simulink model "mrac_sim"  (R2023b)
settings: Solver=VariableStepAuto  StartTime=0.0  StopTime=2200  FixedStep=0.1  RelTol=1e-3  EnableMultiTasking=on
settings Model: Creator=Admin  LastModifiedBy=andre
settings SolverCC: AlgebraicLoopSolver=TrustRegion
settings DataIOCC: LimitDataPoints=on  SaveFormat=Array  ReturnWorkspaceOutputs=off
settings OptimizationCC: ReuseModelBlockBuffer=off  LifeSpan=inf
settings DebuggingCC: UnconnectedInputMsg=warning  UnconnectedOutputMsg=warning  UnconnectedLineMsg=warning  SFUnexpectedBacktrackingDiag=warning  SFNoUnconditionalDefaultTransitionDiag=warning  SFExecutionAtInitializationDiag=none  ArithmeticOperatorsInVariantConditions=warning
settings HardwareCC: ProdBitPerPointer=32  ProdBitPerSizeT=32  ProdBitPerPtrDiffT=32  ProdLargestAtomicFloat=None  ProdIntDivRoundTo=Undefined  ProdEndianess=Unspecified  ProdWordSize=32  ProdHWDeviceType=32-bit Generic
settings ModelReferenceCC: PropagateSignalLabelsOutOfModel=off
settings SFSimCC: SimUseLocalCustomCode=off  CustomCodeUndefinedFunction=UseInterfaceOnly
settings RTWCC: RTWUseLocalCustomCode=off
settings CodeAppCC: StateflowObjectComments=on
settings GRTTargetCC: TargetLangStandard=C89/C90 (ANSI)
settings ConfigComp: CovMetricSettings=dw  CovSaveCumulativeToWorkspaceVar=on  CovSaveSingleToWorkspaceVar=on  CovExternalEMLEnable=off

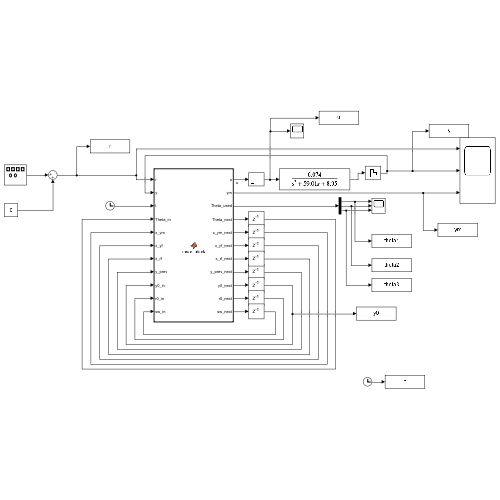
[thumbnail: Simulink's stored preview of the top-level diagram]
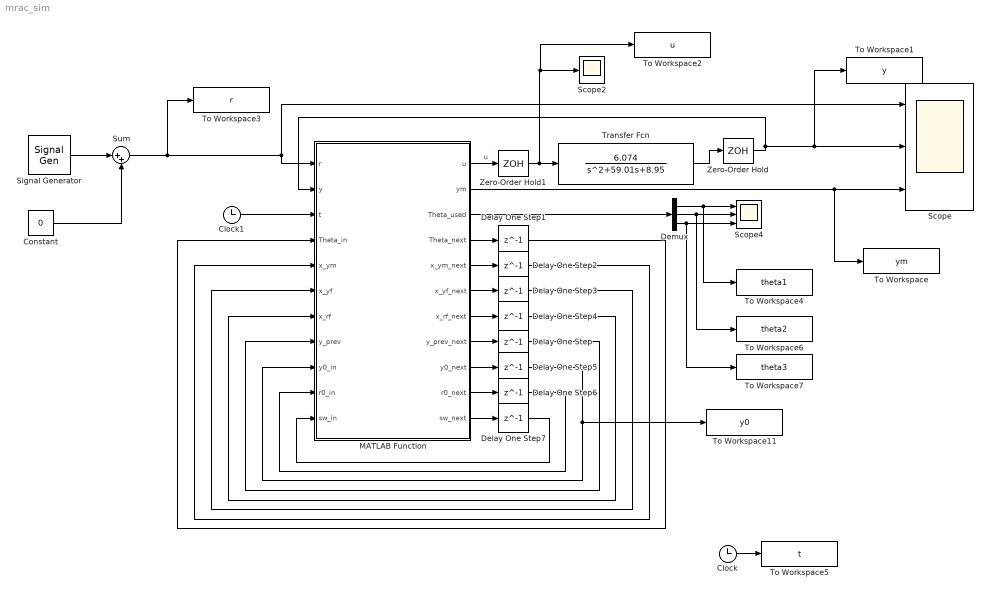
== system mrac_sim ==
  Clock : Clock
  Clock1 : Clock
  Constant : Constant  Value=0
  Delay One Step{,1..7} (8 alike) : Delay  DelayLength=1
  Demux : Demux  Outputs=3
  MATLAB Function : MATLAB Function  TreatAsAtomicUnit=on
  Scope : Scope  NumInputPorts=3
  Scope2 : Scope
  Scope4 : Scope  NumInputPorts=3
  Signal Generator : SignalGenerator  Amplitude=0.5  Frequency=1/400
  Sum : Sum  Inputs=|++
  To Workspace : ToWorkspace  VariableName=ym  SampleTime=0.1
      settings: Save2DSignal=2-D array (concatenate along first dimension)
  To Workspace1 : ToWorkspace  VariableName=y  SampleTime=0.1
      settings: Save2DSignal=2-D array (concatenate along first dimension)
  To Workspace11 : ToWorkspace  VariableName=y0  SampleTime=0.1
      settings: Save2DSignal=2-D array (concatenate along first dimension)
  To Workspace2 : ToWorkspace  VariableName=u  SampleTime=0.1
      settings: Save2DSignal=2-D array (concatenate along first dimension)
  To Workspace3 : ToWorkspace  VariableName=r  SampleTime=0.1
      settings: Save2DSignal=2-D array (concatenate along first dimension)
  To Workspace4 : ToWorkspace  VariableName=theta1  SampleTime=0.1
      settings: Save2DSignal=2-D array (concatenate along first dimension)
  To Workspace5 : ToWorkspace  VariableName=t  SampleTime=0.1
      settings: Save2DSignal=2-D array (concatenate along first dimension)
  To Workspace6 : ToWorkspace  VariableName=theta2  SampleTime=0.1
      settings: Save2DSignal=2-D array (concatenate along first dimension)
  To Workspace7 : ToWorkspace  VariableName=theta3  SampleTime=0.1
      settings: Save2DSignal=2-D array (concatenate along first dimension)
  Transfer Fcn : TransferFcn  Numerator=6.074  Denominator=[1 59.01 8.95]
  Zero-Order Hold : ZeroOrderHold  SampleTime=0.1
  Zero-Order Hold1 : ZeroOrderHold  SampleTime=0.1
  wires:
  Zero-Order Hold/1 -> MATLAB Function/2(y), To Workspace1/1, Scope/2
  Signal Generator/1 -> Sum/1
  Constant/1 -> Sum/2
  MATLAB Function/2(ym) -> To Workspace/1, Scope/3
  MATLAB Function/1(u) -> Zero-Order Hold1/1  "u"
  MATLAB Function/8(y_prev_next) -> Delay One Step/1
  MATLAB Function/7(x_rf_next) -> Delay One Step4/1
  MATLAB Function/6(x_yf_next) -> Delay One Step3/1
  MATLAB Function/5(x_ym_next) -> Delay One Step2/1
  MATLAB Function/4(Theta_next) -> Delay One Step1/1
  Delay One Step/1 -> MATLAB Function/8(y_prev)
  Delay One Step4/1 -> MATLAB Function/7(x_rf)
  Delay One Step3/1 -> MATLAB Function/6(x_yf)
  Delay One Step2/1 -> MATLAB Function/5(x_ym)
  Delay One Step1/1 -> MATLAB Function/4(Theta_in)
  MATLAB Function/3(Theta_used) -> Demux/1
  Demux/1 -> To Workspace4/1, Scope4/1
  Demux/2 -> To Workspace6/1, Scope4/2
  Demux/3 -> To Workspace7/1, Scope4/3
  Zero-Order Hold1/1 -> To Workspace2/1, Scope2/1, Transfer Fcn/1
  Transfer Fcn/1 -> Zero-Order Hold/1
  Sum/1 -> To Workspace3/1, MATLAB Function/1(r), Scope/1
  Clock/1 -> To Workspace5/1
  MATLAB Function/9(y0_next) -> Delay One Step5/1
  MATLAB Function/10(r0_next) -> Delay One Step6/1
  MATLAB Function/11(sw_next) -> Delay One Step7/1
  Delay One Step5/1 -> To Workspace11/1, MATLAB Function/9(y0_in)
  Delay One Step6/1 -> MATLAB Function/10(r0_in)
  Delay One Step7/1 -> MATLAB Function/11(sw_in)
  Clock1/1 -> MATLAB Function/3(t)

== matlab function mrac_sim/MATLAB Function ==
  data: r input size=[1 1]; y input size=[1 1]; t input; u output size=[1 1]; ym output size=[1 1]; Theta_used output size=[3 1]; Theta_in input size=[3 1]; x_ym input size=[2 1]; Theta_next output size=[3 1]; x_yf input size=[2 1]; x_rf input size=[2 1]; y_prev input size=[1 1]; x_ym_next output size=[2 1]; x_yf_next output size=[2 1]; x_rf_next output size=[2 1]; y_prev_next output size=[1 1]; y0_in input; r0_in input; sw_in input; y0_next output; r0_next output; sw_next output
function [u, ym, Theta_used, Theta_next, x_ym_next, x_yf_next, x_rf_next, y_prev_next, y0_next, r0_next, sw_next] = ...
    mrac_block(r, y, t, Theta_in, x_ym, x_yf, x_rf, y_prev, y0_in, r0_in, sw_in)

%params
a0m = 1;
a1m = 20;
b0m = 1;

alpha1 = 14 * 0.01;
alpha2 = 30 * 0.01;
alpha3 = 14 * 0.01;

sign_b0 = 1;
Ts = 0.1;

u0 = 3;
T_settle = 400;

u_min = 0;
u_max = 10;

%State space matrices
A = [0, 1;
    -a0m, -a1m];

b = [0;
    1];

C_yf = [1, 0;
        0, 1];

C_rf = [1, 0];

C_ym = [b0m, 0];

%---
Theta = Theta_in;
Theta_used = Theta;

y0_next = y0_in;
r0_next = r0_in;
sw_next = sw_in;

%---
u = u0;
ym = 0;

Theta_next = Theta;
x_ym_next = x_ym;
x_yf_next = x_yf;
x_rf_next = x_rf;
y_prev_next = y;

%Plant settle

if t < T_settle
    u = u0;
    ym = 0;

    Theta_next = Theta;
    x_ym_next = x_ym;
    x_yf_next = x_yf;
    x_rf_next = x_rf;
    y_prev_next = y;
    y0_next = y0_in;
    r0_next = r0_in;
    sw_next = sw_in;

    return;
end

% transition
if sw_in < 0.5
    y0_next = y;
    r0_next = r;

    x_ym_work = [0; 0];
    x_yf_work = [0; 0];
    x_rf_work = [0; 0];

    Theta_work = Theta;

    y_prev_tilde = 0;
    sw_next = 1;
else
    x_ym_work = x_ym;
    x_yf_work = x_yf;
    x_rf_work = x_rf;

    Theta_work = Theta;

    y_prev_tilde = y_prev - y0_in;
end

% Normalize
y_tilde = y - y0_next;
r_tilde = r - r0_next;

%deriv
ydot_tilde = (y_tilde - y_prev_tilde) / Ts;

%output
ym = C_ym * x_ym_work;
yf_full = C_yf * x_yf_work;
yf = yf_full(1);
ydot_f = yf_full(2);
rf = C_rf * x_rf_work;

%error
e = y_tilde - ym;

omega = [y_tilde; ydot_tilde; r_tilde];

u_tilde = Theta_work.' * omega;
u_unsat = u0 + u_tilde;
u = min(max(u_unsat, u_min), u_max);

%adapt law
dTheta = -sign_b0*e*[alpha1 * yf;
                     alpha2 * ydot_f;
                     alpha3 * rf];

Theta_next = Theta_work + dTheta * Ts;
Theta_used = Theta_work;

%State updates
x_ym_next = x_ym_work + Ts * (A * x_ym_work + b * r_tilde);
x_yf_next = x_yf_work + Ts * (A * x_yf_work + b * y_tilde);
x_rf_next = x_rf_work + Ts * (A * x_rf_work + b * r_tilde);

y_prev_next = y;
